simulink model "test2_11"  (Simulink 7.7)
settings: Solver=ode23  SolverMode=SingleTasking  StartTime=0.0  StopTime=10  MaxStep=1e-4  RelTol=1e-3
libraries: powerlib x12, powerlib_meascontrol x3, pe_lib x1
settings Model: Creator=narendra  LastModifiedBy=narendra  CovMetricSettings=dwe  CovHtmlReporting=off  covSaveCumulativeToWorkspaceVar=off  CovSaveSingleToWorkspaceVar=off  CovExternalEMLEnable=on
settings DataIOCC: LimitDataPoints=off  SaveFormat=StructureWithTime  SignalLoggingSaveFormat=Dataset
settings OptimizationCC: ExpressionDepthLimit=128
settings DebuggingCC: UnderspecifiedInitializationDetection=Simplified  MergeDetectMultiDrivingBlocksExec=error  SolverPrmCheckMsg=none  FcnCallInpInsideContextMsg=Enable All  StateNameClashWarn=none  SFUnexpectedBacktrackingDiag=error  SFNoUnconditionalDefaultTransitionDiag=error
settings HardwareCC: ProdBitPerPointer=64  ProdLargestAtomicFloat=Float  ProdIntDivRoundTo=Zero  ProdEndianess=LittleEndian  ProdHWDeviceType=Specified
settings CodeAppCC: CustomSymbolStrType=$N$R$M_T
settings GRTTargetCC: TargetFunctionLibrary=C99 (ISO)  GeneratePreprocessorConditionals=Use local settings

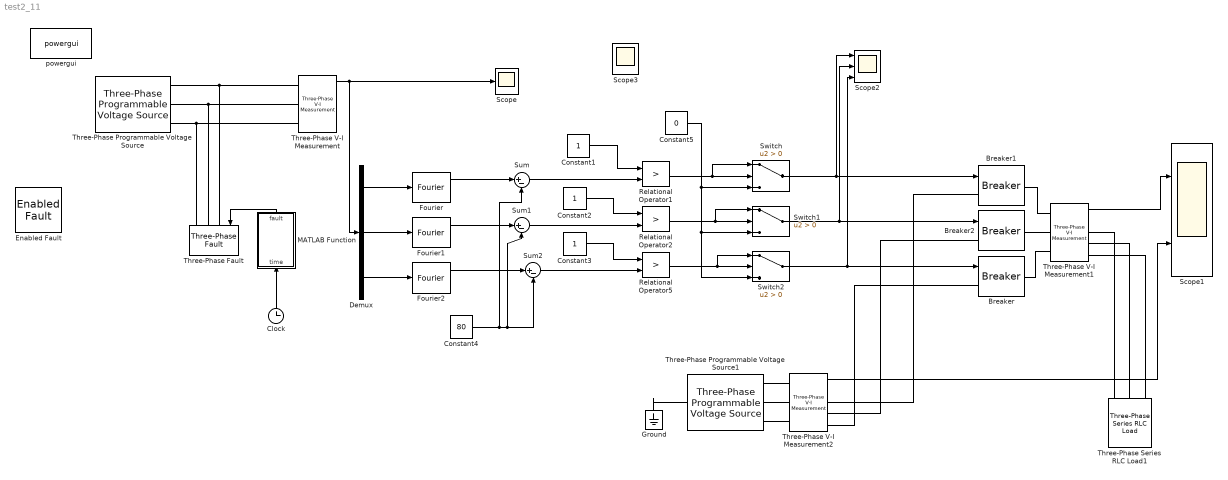
== system test2_11 ==
  Breaker : powerlib/Elements/Breaker  InitialState=0  SwitchingTimes="[1/60  5/60]"  External=on  BreakerResistance=0.01  SnubberResistance=1e6  SnubberCapacitance=inf  Measurements=None  MoreParameters=on  NoBreakLoop=off
  Breaker1 : powerlib/Elements/Breaker  InitialState=0  SwitchingTimes="[1/60  5/60]"  External=on  BreakerResistance=0.01  SnubberResistance=1e6  SnubberCapacitance=inf  Measurements=None  MoreParameters=on  NoBreakLoop=off
  Breaker2 : powerlib/Elements/Breaker  InitialState=0  SwitchingTimes="[1/60  5/60]"  External=on  BreakerResistance=0.01  SnubberResistance=1e6  SnubberCapacitance=inf  Measurements=None  MoreParameters=on  NoBreakLoop=off
  Clock : Clock
  Constant1 : Constant
  Constant2 : Constant
  Constant3 : Constant
  Constant4 : Constant  Value=80
  Constant5 : Constant  Value=0
  Demux : Demux  Outputs=3
  Enabled Fault : pe_lib/Passive Devices/Faults/Enabled Fault  fault_type_option=1  R_pn_fault=1e-3 Ohm  R_ng_fault=1e-3 Ohm  G_parasitic=1e-6 1/Ohm  threshold=0  R_pn_nofault=1e6 Ohm  G_ng_fault=1e3 1/Ohm
  Fourier : powerlib_meascontrol/Measurements/Fourier  Freq=50  n=1  InInit=[0, 0]  Ts=0
  Fourier1 : powerlib_meascontrol/Measurements/Fourier  Freq=50  n=1  InInit=[0, 0]  Ts=0
  Fourier2 : powerlib_meascontrol/Measurements/Fourier  Freq=50  n=1  InInit=[0, 0]  Ts=0
  Ground : powerlib/Elements/Ground  LConnTagsString=a
  MATLAB Function : Stateflow chart  TreatAsAtomicUnit=on
      settings: PermitHierarchicalResolution=ParametersOnly
  Relational Operator1 : RelationalOperator  Operator=>  OutDataTypeStr=boolean
  Relational Operator2 : RelationalOperator  Operator=>  OutDataTypeStr=boolean
  Relational Operator5 : RelationalOperator  Operator=>  OutDataTypeStr=boolean
  Scope : Scope
      settings: TimeRange=5  MaxDataPoints=5000  SaveToWorkspace=off  SaveName=ScopeData  YMin=-168.40242  YMax=168.40242  SampleTime=-1
  Scope1 : Scope  NumInputPorts=2
      settings: TimeRange=10  MaxDataPoints=5000  SaveToWorkspace=off  YMin=-112.26828~-112.26828  YMax=112.26828~112.26828  SampleTime=-1
  Scope2 : Scope  NumInputPorts=3
      settings: TimeRange=auto  MaxDataPoints=5000  SaveToWorkspace=off  SaveName=ScopeData2  YMin=-0.125~-0.125~-0.125  YMax=1.125~1.125~1.125  SampleTime=-1
  Scope3 : Scope
      settings: TimeRange=auto  MaxDataPoints=5000  SaveToWorkspace=off  SaveName=ScopeData3  YMin=-0.125  YMax=1.125  SampleTime=-1
  Sum : Sum  Inputs=|+-
  Sum1 : Sum  Inputs=|+-
  Sum2 : Sum  Inputs=|+-
  Switch : Switch  Criteria=u2 > Threshold  ZeroCross=off
  Switch1 : Switch  Criteria=u2 > Threshold  ZeroCross=off
  Switch2 : Switch  Criteria=u2 > Threshold  ZeroCross=off
  Three-Phase Programmable Voltage Source : powerlib/Electrical Sources/Three-Phase Programmable Voltage Source  PositiveSequence="[110  0 50]"  VariationEntity=None  VariationType=Table of time-amplitude pairs  VariationTypeAlt=Step  VariationStep=0.5  VariationRate=10  VariationMagnitude=0.3  VariationFrequency=2  VariationTiming=[1 2]  VariationPhaseA=off  Amplitudes=[1 0.8 1.2 1.0]  TimeValues=[0 0.1 0.15 0.2]  HarmonicGeneration=off  HarmonicA=[3 0.2 -25 0]  HarmonicB=[2 0.15 35 2]  Timing="[0.05  3]"  BusType=swing  Pref=0  Qref=0  Qmin=-inf  Qmax=inf
  Three-Phase Programmable Voltage Source1 : powerlib/Electrical Sources/Three-Phase Programmable Voltage Source  PositiveSequence="[110  0 50]"  VariationEntity=None  VariationType=Table of time-amplitude pairs  VariationTypeAlt=Step  VariationStep=0.5  VariationRate=10  VariationMagnitude=0.3  VariationFrequency=2  VariationTiming=[1 2]  VariationPhaseA=off  Amplitudes=[1 0.8 1.2 1.0]  TimeValues=[0 0.1 0.15 0.2]  HarmonicGeneration=off  HarmonicA=[3 0.2 -25 0]  HarmonicB=[2 0.15 35 2]  Timing="[0.05  3]"  BusType=swing  Pref=0  Qref=0  Qmin=-inf  Qmax=inf
  Three-Phase Series RLC Load1 : powerlib/Elements/Three-Phase Series RLC Load  LConnTagsString=A|B|C  Configuration=Y (grounded)  NominalVoltage=1000  Vabc=[1e3 1e3 1e3]  Vabcp=[1e3 1e3 1e3]  NominalFrequency=60  UnbalancedPower=off  ActivePower=10e3  InductivePower=100  CapacitivePower=100  Pabc=[10e3 9e3 11e3]  QLabc=[100 90 110]  QCabc=[100 90 110]  Pabcp=[10e3 9e3 11e3]  QLabcp=[100 90 110]  QCabcp=[100 90 110]  Measurements=None  LoadType=constant Z
  Three-Phase V-I Measurement : powerlib/Measurements/Three-Phase V-I Measurement  VoltageMeasurement=phase-to-ground  SetLabelV=off  LabelV=Vabc  Vpu=off  VpuLL=off  CurrentMeasurement=yes  SetLabelI=off  LabelI=Iabc  Ipu=off  Pbase=100e6  Vbase=500e3  OutputType=Complex  PhasorSimulation=off  PSBequivalent=0
  Three-Phase V-I Measurement1 : powerlib/Measurements/Three-Phase V-I Measurement  VoltageMeasurement=phase-to-ground  SetLabelV=off  LabelV=Vabc  Vpu=off  VpuLL=off  CurrentMeasurement=yes  SetLabelI=off  LabelI=Iabc  Ipu=off  Pbase=100e6  Vbase=500e3  OutputType=Complex  PhasorSimulation=off  PSBequivalent=0
  Three-Phase V-I Measurement2 : powerlib/Measurements/Three-Phase V-I Measurement  VoltageMeasurement=phase-to-ground  SetLabelV=off  LabelV=Vabc  Vpu=off  VpuLL=off  CurrentMeasurement=yes  SetLabelI=off  LabelI=Iabc  Ipu=off  Pbase=100e6  Vbase=500e3  OutputType=Complex  PhasorSimulation=off  PSBequivalent=0
  Three-Phase Fault : powerlib/Elements/Three-Phase Fault  InitialStates=[0 0 0]  FaultA=on  FaultB=on  FaultC=off  GroundFault=on  SwitchTimes="[1/60  5/60]"  External=on  SwitchStatus=NaN  FaultResistance=0.0001  GroundResistance=0.001  SnubberResistance=inf  SnubberCapacitance=0  Measurements=Fault voltages
  powergui : powerlib/powergui  Priority=1  SimulationMode=Continuous  SampleTime=50e-6  frequency=50  Iterations=50  frequencyindice=50  Pbase=100e6  ErrMax=1e-4  UnitsV=kV  UnitsW=MW  buscounter=0  FunctionMessages=off  echomessages=off  EnableUseOfTLC=off  CurrentSourceSwitches=off  DisableSnubberDevices=off  DisableRonSwitches=off  DisableVfSwitches=off  DisplayEquations=off  SolverType=Tustin/Backward Euler (TBE)  Interpol=off  ExternalGateDelay=off  methode=off  Ts=100  x0status=blocks  SPID=off  SwTol=0  HookPort=off  RestoreLinks=warning  ResistiveCurrentMeasurement=off  Frange=[0:2:500]  Ylog=off  Xlog=on  ShowGrid=off  save=off  variable=ZData  structure=0  ZoomFFT=off  StartTime=0.0  cycles=1  DisplayStyle=1  fundamental=60  FreqAxis=off  MaxFrequency=1000  frequencyindicesteady=1  RmsSteady=1  display=off
  wires:
  Clock/1 -> MATLAB Function/1(time)
  MATLAB Function/1(fault) -> Three-Phase Fault/1
  Three-Phase V-I Measurement/1 -> Scope/1, Demux/1
  Demux/1 -> Fourier/1
  Demux/2 -> Fourier1/1
  Demux/3 -> Fourier2/1
  Constant1/1 -> Relational Operator1/1
  Constant2/1 -> Relational Operator2/1
  Constant3/1 -> Relational Operator5/1
  Sum/1 -> Relational Operator1/2
  Sum1/1 -> Relational Operator2/2
  Sum2/1 -> Relational Operator5/2
  Constant4/1 -> Sum/2, Sum2/2, Sum1/2
  Fourier/1 -> Sum/1
  Fourier1/1 -> Sum1/1
  Fourier2/1 -> Sum2/1
  Relational Operator1/1 -> Switch/1, Switch/2
  Constant5/1 -> Switch1/3, Switch2/3, Switch/3
  Relational Operator2/1 -> Switch1/1, Switch1/2
  Relational Operator5/1 -> Switch2/1, Switch2/2
  Switch/1 -> Breaker1/1, Scope2/1
  Switch1/1 -> Breaker2/1, Scope2/2
  Switch2/1 -> Breaker/1, Scope2/3
  Three-Phase V-I Measurement1/1 -> Scope1/1
  Three-Phase V-I Measurement2/1 -> Scope1/2
  connections:
  Three-Phase V-I Measurement/LConn1 -- Three-Phase Programmable Voltage Source/RConn1 -- Three-Phase Fault/LConn1
  Three-Phase V-I Measurement/LConn2 -- Three-Phase Programmable Voltage Source/RConn2 -- Three-Phase Fault/LConn2
  Three-Phase V-I Measurement/LConn3 -- Three-Phase Programmable Voltage Source/RConn3 -- Three-Phase Fault/LConn3
  Ground/LConn1 -- Three-Phase Programmable Voltage Source1/LConn1
  Breaker/RConn1 -- Three-Phase V-I Measurement1/LConn3
  Breaker2/RConn1 -- Three-Phase V-I Measurement1/LConn2
  Breaker1/RConn1 -- Three-Phase V-I Measurement1/LConn1
  Three-Phase V-I Measurement2/LConn3 -- Three-Phase Programmable Voltage Source1/RConn3
  Three-Phase V-I Measurement2/LConn2 -- Three-Phase Programmable Voltage Source1/RConn2
  Three-Phase V-I Measurement2/LConn1 -- Three-Phase Programmable Voltage Source1/RConn1
  Three-Phase V-I Measurement2/RConn1 -- Breaker1/LConn1
  Three-Phase V-I Measurement2/RConn2 -- Breaker2/LConn1
  Three-Phase V-I Measurement2/RConn3 -- Breaker/LConn1
  Three-Phase V-I Measurement1/RConn1 -- Three-Phase Series RLC Load1/LConn1
  Three-Phase V-I Measurement1/RConn2 -- Three-Phase Series RLC Load1/LConn2
  Three-Phase V-I Measurement1/RConn3 -- Three-Phase Series RLC Load1/LConn3

== matlab function MATLAB Function ==
  data: time input double; fault output double
function fault = fcn(time)

fault = 0;
if (time<4 && time>2);
    fault=1;
end
